simulink model "SF012A_HysCmp"  (R2013b)
settings: Solver=FixedStepDiscrete  StartTime=0.0  StopTime=1  FixedStep=.002  RelTol=1e-3
values from neighbouring files (symbols this model uses):
  ARCHGLBPRM_2MILLISEC_SEC_F32 = DataDict.Constant    [SF012A_HysCmp_DataDict.m]
  EPSILON_ULS_F32 = DataDict.Constant    [SF012A_HysCmp_DataDict.m]
  FLTINJ_HYSCMP_HYSCMPCMD = DataDict.Constant    [SF012A_HysCmp_DataDict.m]
  HysCmpAssiInpLim = DataDict.Calibration    [SF012A_HysCmp_DataDict.m]
  HysCmpOutpLim = DataDict.Calibration    [SF012A_HysCmp_DataDict.m]
  HysCmpRevGain = DataDict.Calibration    [SF012A_HysCmp_DataDict.m]
  HysCmpRiseX = DataDict.Calibration    [SF012A_HysCmp_DataDict.m]
  HysCmpRiseY = DataDict.Calibration    [SF012A_HysCmp_DataDict.m]
  HYSRISEYLIM_ULS_F32 = DataDict.Constant    [SF012A_HysCmp_DataDict.m]
  HYSSATNLOWLIM_HWNWTMTR_F32 = DataDict.Constant    [SF012A_HysCmp_DataDict.m]
  SysGlbPrmSysTqRat = DataDict.ImprtdCal    [SF012A_HysCmp_DataDict.m]
libraries: FixdToFloat x18, FloatToFixd x14, LnrIntrpn x12, NxtrAbslt x10, NxtrLim x8, Fil x6, NxtrSign x5, simulink x2, NxtrMath x1, BilnrIntrpnMplX x1, NxtrMax x1
(part 2 of 2)

== system SF012A_HysCmp/HysCmp/HysCmpPer1/FilHysCmpOutp/CopyRight2 ==

== system SF012A_HysCmp/HysCmp/HysCmpPer1/FilHysCmpOutp/HysCmp ==
  LpFilSts : Inport
  Action Port : ActionPort  ActionType=else
  Constant1 : Constant  Value=SysGlbPrmSysTqRat
  Constant2 : Constant  Value=HysCmpOutpLim
  CopyRight2 : Subsystem  Description=|  mask(Copyright Information){none=on}
      | Copyright info block.                                               
      |                                                                     
      | Place copyright information at the top of every subsystem in design.
      mask prompts: none "No parameters"
      mask help: Place copyright information at the top of every subsystem in design.
      mask Display:
      | NxtrConf = 'Nexteer Confidential';
      | 
      | sys = bdroot; %handle for the current model ("system")
      | first = get_param(sys,'Created');
      | if(isempty(first))
      |     first = datestr(now,'yyyy');
      | else
      |     first = first(end-3:end);  %year is last four digits
      | end
      | 
      | last = get_param(sys,'LastModifiedDate');
      | if isempty(last)
      |     last = datestr(now,'yyyy');
      | else
      |     last = last(end-3:end);
      | end
      | 
      | if strcmp(first,last)
      |     fprintf('%s -- Copyright %s Nexteer',NxtrConf,first)
      | else
      |     fprintf('%s -- %s%s- %s Nexteer',NxtrConf,char(169),first,last)
      | end
  FinalLim : NxtrLim/LimDyn_f32
  Product : Product  Inputs=*/  RndMeth=Zero
  Unary Minus2 : UnaryMinus
  Out : Outport
  wires:
  LpFilSts/1 -> FinalLim/1
  Unary Minus2/1 -> FinalLim/2
  Constant2/1 -> FinalLim/3, Unary Minus2/1
  FinalLim/1 -> Product/1
  Constant1/1 -> Product/2
  Product/1 -> Out/1

== system SF012A_HysCmp/HysCmp/HysCmpPer1/FilHysCmpOutp/Zero_Command ==
  Action Port : ActionPort  ActionType=then
  Constant1 : Constant  RequirementInfo={} %GIDa_058d0f85_193c_4c5a_9e4f_6786860596fd  Value=0  OutDataTypeStr=single
  CopyRight2 : Subsystem  Description=|  mask(Copyright Information){none=on}
      | Copyright info block.                                               
      |                                                                     
      | Place copyright information at the top of every subsystem in design.
      mask prompts: none "No parameters"
      mask help: Place copyright information at the top of every subsystem in design.
      mask Display:
      | NxtrConf = 'Nexteer Confidential';
      | 
      | sys = bdroot; %handle for the current model ("system")
      | first = get_param(sys,'Created');
      | if(isempty(first))
      |     first = datestr(now,'yyyy');
      | else
      |     first = first(end-3:end);  %year is last four digits
      | end
      | 
      | last = get_param(sys,'LastModifiedDate');
      | if isempty(last)
      |     last = datestr(now,'yyyy');
      | else
      |     last = last(end-3:end);
      | end
      | 
      | if strcmp(first,last)
      |     fprintf('%s -- Copyright %s Nexteer',NxtrConf,first)
      | else
      |     fprintf('%s -- %s%s- %s Nexteer',NxtrConf,char(169),first,last)
      | end
  Out : Outport
  wires:
  Constant1/1 -> Out/1

== system SF012A_HysCmp/HysCmp/HysCmpPer1/FltInj - Sim/CopyRight2 ==

== system SF012A_HysCmp/HysCmp/HysCmpPer1/CalcAvlCmp/CoulombFric/CopyRight2 ==

== system SF012A_HysCmp/HysCmp/HysCmpPer1/CalcRiseFac/LessCmp/CopyRight2 ==

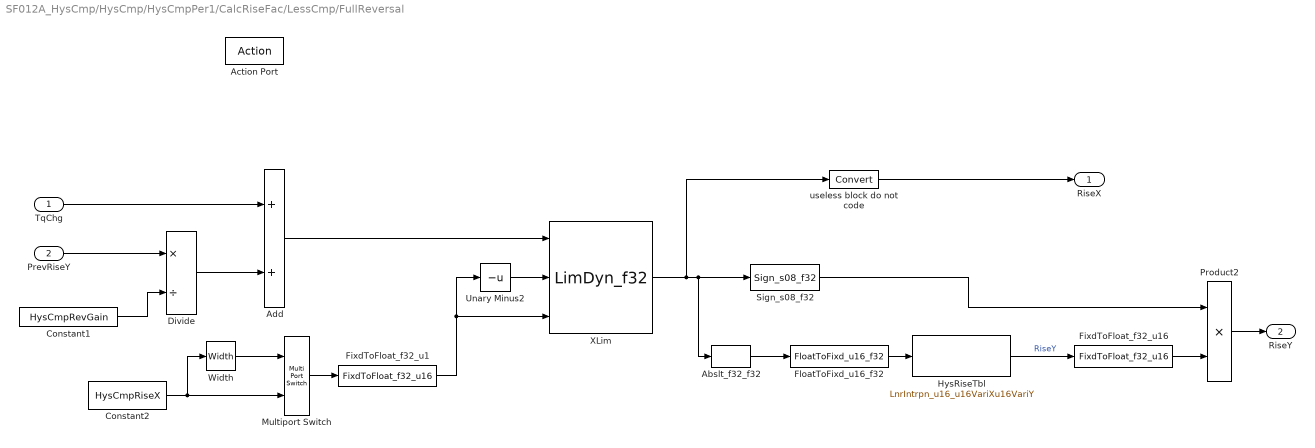
== system SF012A_HysCmp/HysCmp/HysCmpPer1/CalcRiseFac/LessCmp/FullReversal ==
  TqChg : Inport
  PrevRiseY : Inport  Port=2
  Action Port : ActionPort  ActionType=else
  Abslt_f32_f32 : NxtrAbslt/Abslt_f32_f32  SFunctionSpec=single y1 = Abslt_f32_f32(single u1)
      settings: AttributesFormatString=%<Name>
  Add : Sum  RndMeth=Zero
  Constant1 : Constant  Value=HysCmpRevGain
  Constant2 : Constant  Value=HysCmpRiseX
  Divide : Product  Inputs=*/  RndMeth=Zero
  FixdToFloat_f32_u1 : FixdToFloat/FixdToFloat_f32_u16  Param1=14
  FixdToFloat_f32_u16 : FixdToFloat/FixdToFloat_f32_u16  Param1=14
  FloatToFixd_u16_f32 : FloatToFixd/FloatToFixd_u16_f32  Param1=14
  HysRiseTbl : LnrIntrpn/LnrIntrpn_u16_u16VariXu16VariY  XTbl=HysCmpRiseX  YTbl=HysCmpRiseY
      settings: AttributesFormatString=Lnr ( u16VariX , u16VariY )
  Multiport Switch : MultiPortSwitch  Inputs=1
  Product2 : Product  RndMeth=Zero
  Sign_s08_f32 : NxtrSign/Sign_s08_f32  SFunctionSpec=int8 y1 = Sign_s08_f32(single u1)
  Unary Minus2 : UnaryMinus
  Width : Width  DataType=uint16
  XLim : NxtrLim/LimDyn_f32
  useless block do not code : DataTypeConversion
  RiseX : Outport
  RiseY : Outport  Port=2
  wires:
  Constant1/1 -> Divide/2
  PrevRiseY/1 -> Divide/1
  Divide/1 -> Add/2
  TqChg/1 -> Add/1
  Add/1 -> XLim/1
  FixdToFloat_f32_u1/1 -> XLim/3, Unary Minus2/1
  Unary Minus2/1 -> XLim/2
  XLim/1 -> Abslt_f32_f32/1, Sign_s08_f32/1, useless block do not code/1
  HysRiseTbl/1 -> FixdToFloat_f32_u16/1  "RiseY"
  Abslt_f32_f32/1 -> FloatToFixd_u16_f32/1
  Sign_s08_f32/1 -> Product2/1
  Product2/1 -> RiseY/1
  FixdToFloat_f32_u16/1 -> Product2/2
  FloatToFixd_u16_f32/1 -> HysRiseTbl/1
  Constant2/1 -> Multiport Switch/2, Width/1
  Width/1 -> Multiport Switch/1
  Multiport Switch/1 -> FixdToFloat_f32_u1/1
  useless block do not code/1 -> RiseX/1

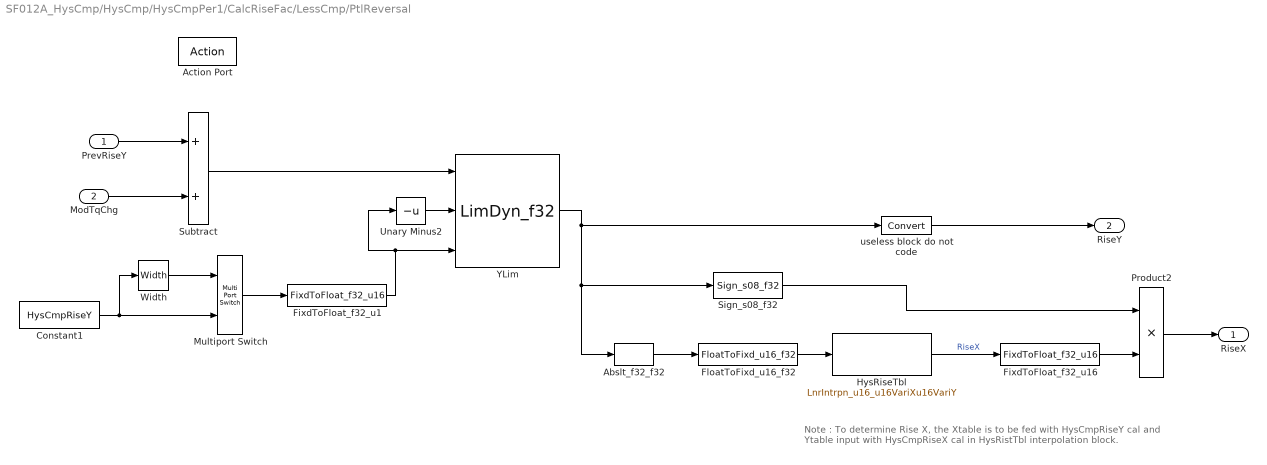
== system SF012A_HysCmp/HysCmp/HysCmpPer1/CalcRiseFac/LessCmp/PtlReversal ==
  note: Note : To determine Rise X, the Xtable is to be fed with HysCmpRiseY cal
      | and Ytable input with HysCmpRiseX cal in HysRistTbl interpolation block.
  PrevRiseY : Inport
  ModTqChg : Inport  Port=2
  Action Port : ActionPort  ActionType=then
  Abslt_f32_f32 : NxtrAbslt/Abslt_f32_f32  SFunctionSpec=single y1 = Abslt_f32_f32(single u1)
      settings: AttributesFormatString=%<Name>
  Constant1 : Constant  Value=HysCmpRiseY
  FixdToFloat_f32_u1 : FixdToFloat/FixdToFloat_f32_u16  Param1=14
  FixdToFloat_f32_u16 : FixdToFloat/FixdToFloat_f32_u16  Param1=14
  FloatToFixd_u16_f32 : FloatToFixd/FloatToFixd_u16_f32  Param1=14
  HysRiseTbl : LnrIntrpn/LnrIntrpn_u16_u16VariXu16VariY  XTbl=HysCmpRiseY  YTbl=HysCmpRiseX
      settings: AttributesFormatString=Lnr ( u16VariX , u16VariY )
  Multiport Switch : MultiPortSwitch  Inputs=1
  Product2 : Product  RndMeth=Zero
  Sign_s08_f32 : NxtrSign/Sign_s08_f32  SFunctionSpec=int8 y1 = Sign_s08_f32(single u1)
  Subtract : Sum  RndMeth=Zero
  Unary Minus2 : UnaryMinus
  Width : Width  DataType=uint16
  YLim : NxtrLim/LimDyn_f32
  useless block do not code : DataTypeConversion
  RiseX : Outport
  RiseY : Outport  Port=2
  wires:
  PrevRiseY/1 -> Subtract/1
  ModTqChg/1 -> Subtract/2
  Subtract/1 -> YLim/1
  Unary Minus2/1 -> YLim/2
  YLim/1 -> Abslt_f32_f32/1, Sign_s08_f32/1, useless block do not code/1
  HysRiseTbl/1 -> FixdToFloat_f32_u16/1  "RiseX"
  Abslt_f32_f32/1 -> FloatToFixd_u16_f32/1
  Sign_s08_f32/1 -> Product2/1
  FloatToFixd_u16_f32/1 -> HysRiseTbl/1
  Product2/1 -> RiseX/1
  FixdToFloat_f32_u16/1 -> Product2/2
  Constant1/1 -> Multiport Switch/2, Width/1
  Width/1 -> Multiport Switch/1
  Multiport Switch/1 -> FixdToFloat_f32_u1/1
  FixdToFloat_f32_u1/1 -> Unary Minus2/1, YLim/3
  useless block do not code/1 -> RiseY/1

== system SF012A_HysCmp/HysCmp/HysCmpPer1/CalcRiseFac/MoreCmp/CopyRight2 ==

== system SF012A_HysCmp/HysCmp/HysCmpPer1/CalcRiseFac/NoChg/CopyRight2 ==

== system SF012A_HysCmp/HysCmp/HysCmpPer1/FilAndLimInp/If Action Subsystem/CopyRight2 ==

== system SF012A_HysCmp/HysCmp/HysCmpPer1/FilAndLimInp/If Action Subsystem1/CopyRight2 ==

== system SF012A_HysCmp/HysCmp/HysCmpPer1/FilHysCmpOutp/HysCmp/CopyRight2 ==

== system SF012A_HysCmp/HysCmp/HysCmpPer1/FilHysCmpOutp/Zero_Command/CopyRight2 ==
